simulink model "Lab_4"  (R2019b)
settings: Solver=ode23  StartTime=0.0  StopTime=50  MaxStep=0.02  RelTol=1e-6  AbsTol=1e-6
model workspace (MATLAB code in the model file):
  | %% Variable
  | s = tf('s');
  | 
  | %% Generate Plant Linearization
  | LinearPlant = 1/(s^2);
values from neighbouring files (symbols this model uses):
  filterCoeff = 100.0    [Lab_4_Data.sldd]
  pathDirection = 1.0 2.0    [Lab_4_Data.sldd]
  pathReferencePoint = 0.0 0.0    [Lab_4_Data.sldd]
  V = 40.0    [Lab_4_Data.sldd]
  windRadial = 270.0    [Lab_4_Data.sldd]
  windSpeed = 15.0    [Lab_4_Data.sldd]
  x0 = 0.0 0.0 1.285    [Lab_4_Data.sldd]
libraries: dspmathops x2, simulink x1
settings Model: DataDictionary=Lab_4_Data.sldd  Creator=rolle  LastModifiedBy=Arjun
settings SolverCC: ZeroCrossAlgorithm=Adaptive
settings DataIOCC: SaveOutput=off  DSMLogging=off  SaveTime=off  ReturnWorkspaceOutputs=off
settings DebuggingCC: IgnoredZcDiagnostic=none

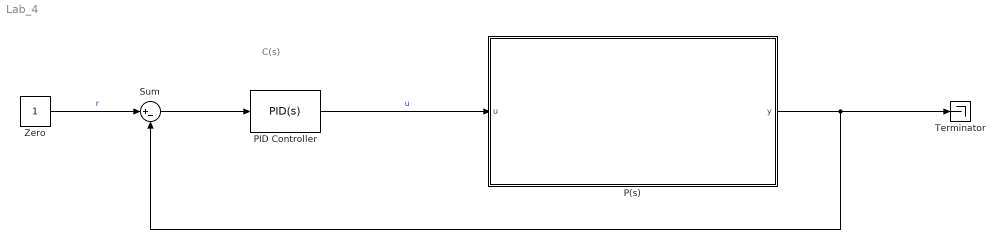
== system Lab_4 ==
  note: C(s)
  P(s) : Subsystem  SCDEnableBlockLinearizationSpecification=on
  PID Controller : simulink/Continuous/PID Controller  Controller=PID  Form=Parallel  TimeDomain=Continuous-time  SampleTime=-1  IntegratorMethod=Forward Euler  FilterMethod=Forward Euler  ControllerParametersSource=internal  P=8  I=20  D=3  UseFilter=on  N=filterCoeff  TunerSelectOption=Transfer Function Based (PID Tuner App)  InitialConditionSource=internal  InitialConditionForIntegrator=0  InitialConditionForFilter=0  DifferentiatorICPrevScaledInput=0  ExternalReset=none  TrackingMode=off  Kt=1  LimitOutput=off  UpperSaturationLimit=pi/30  LowerSaturationLimit=-pi/30  LinearizeAsGain=on  AntiWindupMode=back-calculation  Kb=10  POutMin=[]  POutMax=[]  IOutMin=[]  IOutMax=[]  DOutMin=[]  DOutMax=[]  NOutMin=[]  NOutMax=[]  SumOutMin=[]  SumOutMax=[]  SaturationOutMin=[]  SaturationOutMax=[]  PParamMin=[]  PParamMax=[]  IParamMin=[]  IParamMax=[]  DParamMin=[]  DParamMax=[]  NParamMin=[]  NParamMax=[]  KbParamMin=[]  KbParamMax=[]  KtParamMin=[]  KtParamMax=[]  KbOutMin=[]  KbOutMax=[]  KtOutMin=[]  KtOutMax=[]  IntegratorOutMin=[]  IntegratorOutMax=[]  FilterOutMin=[]  FilterOutMax=[]  SumI1OutMin=[]  SumI1OutMax=[]  SumI2OutMin=[]  SumI2OutMax=[]  SumI3OutMin=[]  SumI3OutMax=[]  SumI4OutMin=[]  SumI4OutMax=[]  SumDOutMin=[]  SumDOutMax=[]  DifferentiatorOutMin=[]  DifferentiatorOutMax=[]  FilterDiffOutCoefMin=[]  FilterDiffOutCoefMax=[]  ReciprocalOutMin=[]  ReciprocalOutMax=[]  SumDenOutMin=[]  SumDenOutMax=[]  SumNumOutMin=[]  SumNumOutMax=[]  DivideOutMin=[]  DivideOutMax=[]  IntegratorContinuousStateAttributes=''  IntegratorStateMustResolveToSignalObject=off  IntegratorRTWStateStorageClass=Auto  FilterContinuousStateAttributes=''  FilterStateMustResolveToSignalObject=off  FilterRTWStateStorageClass=Auto  ParallelPVariant=InternalParameters  IdealPVariant=Disabled  IVariant=InternalParameters  DVariant=InternalParameters  IntegratorVariant=Continuous  SatVariant=Disabled  AWVariant=Passthrough  PCopyVariant=Disabled  TRVariant=Disabled  FdbkBlocksVariant=Forward  IdealPFdbkVariant=Disabled  SatFdbkVariant=Disabled  DerivativeFilterVariant=ContFilter  NVariant=InternalParameters  NCopyVariant=Disabled  FilterICVariant=InternalICsFilter  IntegratorICVariant=InternalICs  ExternalResetVariant=Disabled  TRSumVariant=Passthrough  SumFdbkVariant=Disabled  SumVariant=Sum_PID
  Sum : Sum  Inputs=|+-
  Terminator : Terminator
  Zero : Constant  OutDataTypeStr=Inherit: Inherit via back propagation
  wires:
  Zero/1 -> Sum/1  "r"
  Sum/1 -> PID Controller/1
  P(s)/1(y) -> Sum/2, Terminator/1
  PID Controller/1 -> P(s)/1(u)  "u"

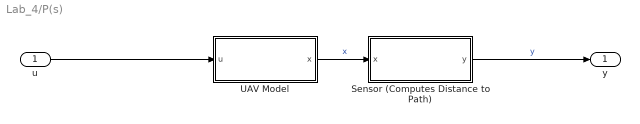
== system Lab_4/P(s) ==
  u : Inport
  Sensor (Computes Distance to Path) : Subsystem
  UAV Model : Subsystem
  y : Outport
  wires:
  UAV Model/1(x) -> Sensor (Computes Distance to Path)/1(x)  "x"
  u/1 -> UAV Model/1(u)
  Sensor (Computes Distance to Path)/1(y) -> y/1  "y"

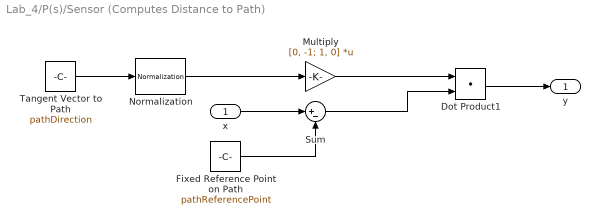
== system Lab_4/P(s)/Sensor (Computes Distance to Path) ==
  x : Inport
  Dot Product1 : DotProduct  InputSameDT=on  OutDataTypeStr=Inherit: Inherit via internal rule
  Fixed Reference Point on Path : Constant  Value=pathReferencePoint
  Multiply : Gain  Gain=[0, -1; 1, 0]  Multiplication=Matrix(K*u)
  Normalization : dspmathops/Normalization  NormType=2-norm  Bias=1e-10  NormOver=Each column  Dimension=1  roundingMode=Floor  overflowMode=off  accumDataTypeStr=Inherit: Same as product output  accumLastDataTypeStr=Inherit: Same as product output  outputDataTypeStr=Inherit: Same as product output  outputMin=[]  outputMax=[]  outputLastDataTypeStr=Inherit: Same as product output
  Sum : Sum  Inputs=|+-
  Tangent Vector to Path : Constant  Value=pathDirection
  y : Outport
  wires:
  Tangent Vector to Path/1 -> Normalization/1
  x/1 -> Sum/1
  Sum/1 -> Dot Product1/2
  Fixed Reference Point on Path/1 -> Sum/2
  Normalization/1 -> Multiply/1
  Dot Product1/1 -> y/1
  Multiply/1 -> Dot Product1/1

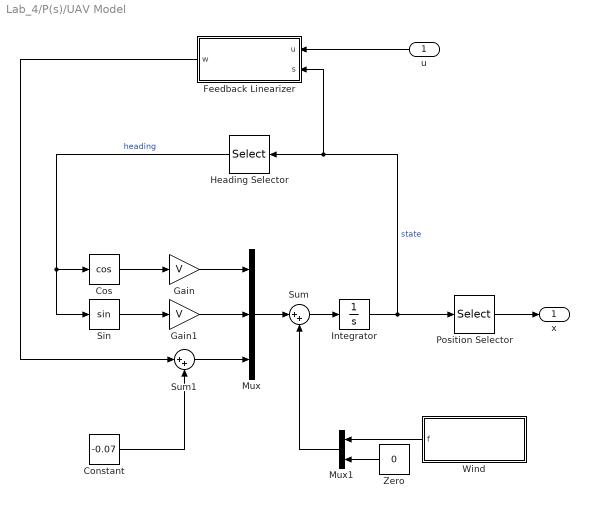
== system Lab_4/P(s)/UAV Model ==
  u : Inport
  Constant : Constant  Value=-0.07
  Cos : Trigonometry  Operator=cos
  Feedback Linearizer : Subsystem
  Gain : Gain  Gain=V
  Gain1 : Gain  Gain=V
  Heading Selector : Selector  InputPortWidth=3  IndexOptions=Index vector (dialog)  Indices=3  OutputSizes=1
  Integrator : Integrator  InitialCondition=x0
  Mux : Mux  Inputs=3
  Mux1 : Mux  Inputs=2
  Position Selector : Selector  InputPortWidth=3  IndexOptions=Index vector (dialog)  Indices=[1 2]  OutputSizes=1
  Sin : Trigonometry
  Sum : Sum  Inputs=|++
  Sum1 : Sum  Inputs=|++
  Wind : Subsystem
  Zero : Constant  Value=0  OutDataTypeStr=Inherit: Inherit via back propagation
  x : Outport
  wires:
  Position Selector/1 -> x/1
  Integrator/1 -> Heading Selector/1, Feedback Linearizer/2(s), Position Selector/1  "state"
  Heading Selector/1 -> Sin/1, Cos/1  "heading"
  Cos/1 -> Gain/1
  Gain/1 -> Mux/1
  Sin/1 -> Gain1/1
  Gain1/1 -> Mux/2
  Mux/1 -> Sum/1
  Sum/1 -> Integrator/1
  Wind/1(f) -> Mux1/1
  Mux1/1 -> Sum/2
  Zero/1 -> Mux1/2
  Sum1/1 -> Mux/3
  Constant/1 -> Sum1/2
  Feedback Linearizer/1(w) -> Sum1/1
  u/1 -> Feedback Linearizer/1(u)

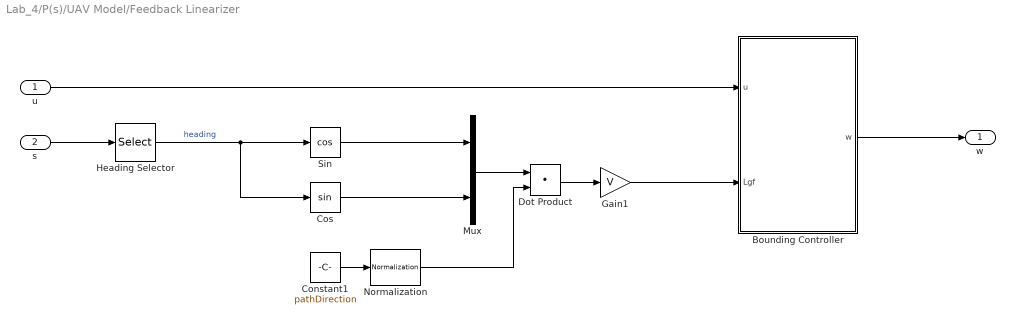
== system Lab_4/P(s)/UAV Model/Feedback Linearizer ==
  u : Inport
  s : Inport  Port=2
  Bounding Controller : MATLAB Function  TreatAsAtomicUnit=on
  Constant1 : Constant  Value=pathDirection
  Cos : Trigonometry
  Dot Product : DotProduct  InputSameDT=on  OutDataTypeStr=Inherit: Inherit via internal rule
  Gain1 : Gain  Gain=V
  Heading Selector : Selector  InputPortWidth=3  IndexOptions=Index vector (dialog)  Indices=3  OutputSizes=1
  Mux : Mux  Inputs=2
  Normalization : dspmathops/Normalization  NormType=2-norm  Bias=1e-10  NormOver=Each column  Dimension=1  roundingMode=Floor  overflowMode=off  accumDataTypeStr=Inherit: Same as product output  accumLastDataTypeStr=Inherit: Same as product output  outputDataTypeStr=Inherit: Same as product output  outputMin=[]  outputMax=[]  outputLastDataTypeStr=Inherit: Same as product output
  Sin : Trigonometry  Operator=cos
  w : Outport
  wires:
  s/1 -> Heading Selector/1
  Heading Selector/1 -> Cos/1, Sin/1  "heading"
  Cos/1 -> Mux/2
  Sin/1 -> Mux/1
  Mux/1 -> Dot Product/1
  Constant1/1 -> Normalization/1
  Dot Product/1 -> Gain1/1
  Bounding Controller/1(w) -> w/1
  Gain1/1 -> Bounding Controller/2(Lgf)
  u/1 -> Bounding Controller/1(u)
  Normalization/1 -> Dot Product/2

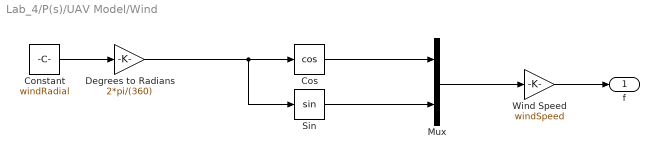
== system Lab_4/P(s)/UAV Model/Wind ==
  Constant : Constant  Value=windRadial
  Cos : Trigonometry  Operator=cos
  Degrees to Radians : Gain  Gain=2*pi/(360)
  Mux : Mux  Inputs=2
  Sin : Trigonometry
  Wind Speed : Gain  Gain=windSpeed
  f : Outport
  wires:
  Wind Speed/1 -> f/1
  Constant/1 -> Degrees to Radians/1
  Cos/1 -> Mux/1
  Sin/1 -> Mux/2
  Mux/1 -> Wind Speed/1
  Degrees to Radians/1 -> Sin/1, Cos/1

== matlab function Lab_4/P(s)/UAV Model/Feedback Linearizer/Bounding Controller ==
  data: u input; w output; Lgf input
function w = Bounding(u, Lgf)
    if abs(Lgf) <= 1e-2
        w = u / (sign(Lgf)*1e-2);        
    else
        w = u / (Lgf);
    end
end
